simulink model "SUB_IoControl"  (R2018b)
settings: Solver=VariableStepDiscrete  StartTime=0.0  StopTime=10  RelTol=1e-3
PreLoadFcn:
  | if(exist('MBDS_ModelCallback', 'file'))
  |    MBDS_ModelCallback('PreLoad');
  | end
PostLoadFcn:
  | if(exist('MBDS_ModelCallback', 'file'))
  |    MBDS_ModelCallback('PostLoad');
  | end
InitFcn:
  | if(exist('MBDS_ModelCallback', 'file'))
  |    MBDS_ModelCallback('Init');
  | end
StartFcn:
  | if(exist('MBDS_ModelCallback', 'file'))
  |    MBDS_ModelCallback('Start');
  | end
StopFcn:
  | if(exist('MBDS_ModelCallback', 'file'))
  |    MBDS_ModelCallback('Stop');
  | end
undefined symbols (not defined in the file): sigbuilder_block
libraries: KIBES_Signal x742, MBDS_Modules x38, simulink x1
(part 2 of 8)

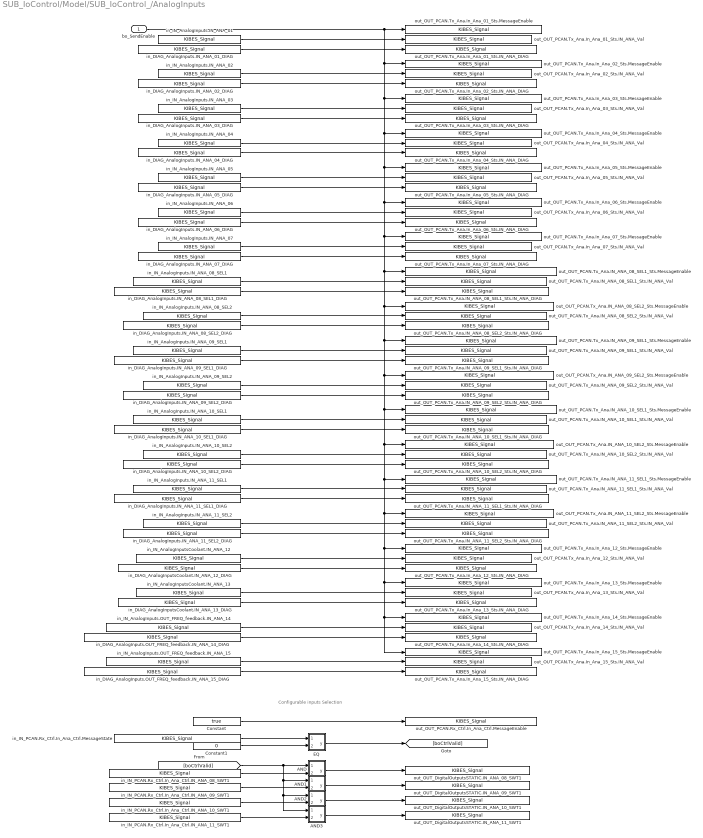
== system SUB_IoControl/Model/SUB_IoControl_/AnalogInputs ==
  note: Configurable inputs Selection
  bo_SendEnable : Inport
  AND : Subsystem  InitFcn=|  mask(AND){MBDS_LibraryBlock=on, BitwiseMode=off, Inputs=2, UseBitMask=off, BitMask='A7', OutDataTypeStr=Inherit: Inherit via back propagation, MBDS_BlockVersion=08.20.02}
      | if(exist('MBDS_BlockCallback', 'file'))
      |    MBDS_BlockCallback('Update', gcb);
      | end
      mask prompts: MBDS_LibraryBlock "MBDS library block"; BitwiseMode "Use 'bitwise' mode"; Inputs "Number of input ports:"; UseBitMask "Use bit mask"; BitMask "Bit mask:"; OutDataTypeStr "Output data type:"; MBDS_BlockVersion "Version:"
      mask help: Logical or bitwise AND operator. For multiple inputs, operators are applied across the inputs. For a single input, operators are applied across the input vector. In bitwise mode a bit mask can be applied onto single input signals.
      mask init: same as SUB_IoControl/Outputs/AnalyseOutputs/And
      mask Help: eval(['open([workdir(''library_dir:''),''\Blockset\help\'',get_param(gcb,''MaskType''),''.html''])'])
      mask Callback BitwiseMode:
      | if(exist('MBDS_BlockCallback', 'file'))
      |    MBDS_BlockCallback('BitwiseMode', gcb);
      | end
      mask Callback Inputs:
      | if(exist('MBDS_BlockCallback', 'file'))
      |    MBDS_BlockCallback('Inputs', gcb);
      | end
      mask Callback UseBitMask:
      | if(exist('MBDS_BlockCallback', 'file'))
      |    MBDS_BlockCallback('UseBitMask', gcb);
      | end
      mask Callback BitMask:
      | if(exist('MBDS_BlockCallback', 'file'))
      |    MBDS_BlockCallback('BitMask', gcb);
      | end
      mask TypeOptions OutDataTypeStr: Inherit: Inherit via back propagation | int8 | uint8 | int16 | uint16 | int32 | uint32 | boolean
      mask Callback OutDataTypeStr:
      | % Adopt Value
      | if(exist('MBDS_BlockCallback', 'file'))
      |    MBDS_BlockCallback('OutDataTypeStr', gcb);
      | end
      mask DialogControl ParameterTabVar0 Prompt: Main
      mask DialogControl ParameterTabVar01 Prompt: Signal Attributes
      mask DialogControl ParameterTabVar012 Prompt: Version
      mask Display:
      | % Show icon or block text
      | if(UseBitMask)
      |    if(isnumeric(BitMask))
      |       BitMaskString = ['0x',dec2hex(floor(BitMask))];
      |    elseif(ischar(BitMask))
      |       BitMaskString = ['0x',upper(BitMask)];
      |    else
      |       BitMaskString = '???';
      |    end
      |    disp(sprintf(['AND\n', BitMaskString]))
      | else
      |    disp('AND')
      | end
  AND1 : Subsystem  InitFcn=|  mask(AND){MBDS_LibraryBlock=on, BitwiseMode=off, Inputs=2, UseBitMask=off, BitMask='A7', OutDataTypeStr=Inherit: Inherit via back propagation, MBDS_BlockVersion=08.20.02}
      | if(exist('MBDS_BlockCallback', 'file'))
      |    MBDS_BlockCallback('Update', gcb);
      | end
      mask prompts: MBDS_LibraryBlock "MBDS library block"; BitwiseMode "Use 'bitwise' mode"; Inputs "Number of input ports:"; UseBitMask "Use bit mask"; BitMask "Bit mask:"; OutDataTypeStr "Output data type:"; MBDS_BlockVersion "Version:"
      mask help: Logical or bitwise AND operator. For multiple inputs, operators are applied across the inputs. For a single input, operators are applied across the input vector. In bitwise mode a bit mask can be applied onto single input signals.
      mask init: same as SUB_IoControl/Outputs/AnalyseOutputs/And
      mask Help: eval(['open([workdir(''library_dir:''),''\Blockset\help\'',get_param(gcb,''MaskType''),''.html''])'])
      mask Callback BitwiseMode:
      | if(exist('MBDS_BlockCallback', 'file'))
      |    MBDS_BlockCallback('BitwiseMode', gcb);
      | end
      mask Callback Inputs:
      | if(exist('MBDS_BlockCallback', 'file'))
      |    MBDS_BlockCallback('Inputs', gcb);
      | end
      mask Callback UseBitMask:
      | if(exist('MBDS_BlockCallback', 'file'))
      |    MBDS_BlockCallback('UseBitMask', gcb);
      | end
      mask Callback BitMask:
      | if(exist('MBDS_BlockCallback', 'file'))
      |    MBDS_BlockCallback('BitMask', gcb);
      | end
      mask TypeOptions OutDataTypeStr: Inherit: Inherit via back propagation | int8 | uint8 | int16 | uint16 | int32 | uint32 | boolean
      mask Callback OutDataTypeStr:
      | % Adopt Value
      | if(exist('MBDS_BlockCallback', 'file'))
      |    MBDS_BlockCallback('OutDataTypeStr', gcb);
      | end
      mask DialogControl ParameterTabVar0 Prompt: Main
      mask DialogControl ParameterTabVar01 Prompt: Signal Attributes
      mask DialogControl ParameterTabVar012 Prompt: Version
      mask Display:
      | % Show icon or block text
      | if(UseBitMask)
      |    if(isnumeric(BitMask))
      |       BitMaskString = ['0x',dec2hex(floor(BitMask))];
      |    elseif(ischar(BitMask))
      |       BitMaskString = ['0x',upper(BitMask)];
      |    else
      |       BitMaskString = '???';
      |    end
      |    disp(sprintf(['AND\n', BitMaskString]))
      | else
      |    disp('AND')
      | end
  AND2 : Subsystem  InitFcn=|  mask(AND){MBDS_LibraryBlock=on, BitwiseMode=off, Inputs=2, UseBitMask=off, BitMask='A7', OutDataTypeStr=Inherit: Inherit via back propagation, MBDS_BlockVersion=08.20.02}
      | if(exist('MBDS_BlockCallback', 'file'))
      |    MBDS_BlockCallback('Update', gcb);
      | end
      mask prompts: MBDS_LibraryBlock "MBDS library block"; BitwiseMode "Use 'bitwise' mode"; Inputs "Number of input ports:"; UseBitMask "Use bit mask"; BitMask "Bit mask:"; OutDataTypeStr "Output data type:"; MBDS_BlockVersion "Version:"
      mask help: Logical or bitwise AND operator. For multiple inputs, operators are applied across the inputs. For a single input, operators are applied across the input vector. In bitwise mode a bit mask can be applied onto single input signals.
      mask init: same as SUB_IoControl/Outputs/AnalyseOutputs/And
      mask Help: eval(['open([workdir(''library_dir:''),''\Blockset\help\'',get_param(gcb,''MaskType''),''.html''])'])
      mask Callback BitwiseMode:
      | if(exist('MBDS_BlockCallback', 'file'))
      |    MBDS_BlockCallback('BitwiseMode', gcb);
      | end
      mask Callback Inputs:
      | if(exist('MBDS_BlockCallback', 'file'))
      |    MBDS_BlockCallback('Inputs', gcb);
      | end
      mask Callback UseBitMask:
      | if(exist('MBDS_BlockCallback', 'file'))
      |    MBDS_BlockCallback('UseBitMask', gcb);
      | end
      mask Callback BitMask:
      | if(exist('MBDS_BlockCallback', 'file'))
      |    MBDS_BlockCallback('BitMask', gcb);
      | end
      mask TypeOptions OutDataTypeStr: Inherit: Inherit via back propagation | int8 | uint8 | int16 | uint16 | int32 | uint32 | boolean
      mask Callback OutDataTypeStr:
      | % Adopt Value
      | if(exist('MBDS_BlockCallback', 'file'))
      |    MBDS_BlockCallback('OutDataTypeStr', gcb);
      | end
      mask DialogControl ParameterTabVar0 Prompt: Main
      mask DialogControl ParameterTabVar01 Prompt: Signal Attributes
      mask DialogControl ParameterTabVar012 Prompt: Version
      mask Display:
      | % Show icon or block text
      | if(UseBitMask)
      |    if(isnumeric(BitMask))
      |       BitMaskString = ['0x',dec2hex(floor(BitMask))];
      |    elseif(ischar(BitMask))
      |       BitMaskString = ['0x',upper(BitMask)];
      |    else
      |       BitMaskString = '???';
      |    end
      |    disp(sprintf(['AND\n', BitMaskString]))
      | else
      |    disp('AND')
      | end
  AND3 : Subsystem  InitFcn=|  mask(AND){MBDS_LibraryBlock=on, BitwiseMode=off, Inputs=2, UseBitMask=off, BitMask='A7', OutDataTypeStr=Inherit: Inherit via back propagation, MBDS_BlockVersion=08.20.02}
      | if(exist('MBDS_BlockCallback', 'file'))
      |    MBDS_BlockCallback('Update', gcb);
      | end
      mask prompts: MBDS_LibraryBlock "MBDS library block"; BitwiseMode "Use 'bitwise' mode"; Inputs "Number of input ports:"; UseBitMask "Use bit mask"; BitMask "Bit mask:"; OutDataTypeStr "Output data type:"; MBDS_BlockVersion "Version:"
      mask help: Logical or bitwise AND operator. For multiple inputs, operators are applied across the inputs. For a single input, operators are applied across the input vector. In bitwise mode a bit mask can be applied onto single input signals.
      mask init: same as SUB_IoControl/Outputs/AnalyseOutputs/And
      mask Help: eval(['open([workdir(''library_dir:''),''\Blockset\help\'',get_param(gcb,''MaskType''),''.html''])'])
      mask Callback BitwiseMode:
      | if(exist('MBDS_BlockCallback', 'file'))
      |    MBDS_BlockCallback('BitwiseMode', gcb);
      | end
      mask Callback Inputs:
      | if(exist('MBDS_BlockCallback', 'file'))
      |    MBDS_BlockCallback('Inputs', gcb);
      | end
      mask Callback UseBitMask:
      | if(exist('MBDS_BlockCallback', 'file'))
      |    MBDS_BlockCallback('UseBitMask', gcb);
      | end
      mask Callback BitMask:
      | if(exist('MBDS_BlockCallback', 'file'))
      |    MBDS_BlockCallback('BitMask', gcb);
      | end
      mask TypeOptions OutDataTypeStr: Inherit: Inherit via back propagation | int8 | uint8 | int16 | uint16 | int32 | uint32 | boolean
      mask Callback OutDataTypeStr:
      | % Adopt Value
      | if(exist('MBDS_BlockCallback', 'file'))
      |    MBDS_BlockCallback('OutDataTypeStr', gcb);
      | end
      mask DialogControl ParameterTabVar0 Prompt: Main
      mask DialogControl ParameterTabVar01 Prompt: Signal Attributes
      mask DialogControl ParameterTabVar012 Prompt: Version
      mask Display:
      | % Show icon or block text
      | if(UseBitMask)
      |    if(isnumeric(BitMask))
      |       BitMaskString = ['0x',dec2hex(floor(BitMask))];
      |    elseif(ischar(BitMask))
      |       BitMaskString = ['0x',upper(BitMask)];
      |    else
      |       BitMaskString = '???';
      |    end
      |    disp(sprintf(['AND\n', BitMaskString]))
      | else
      |    disp('AND')
      | end
  Constant : Constant  InitFcn=|  Value=true  OutDataTypeStr=boolean
      | if(exist('MBDS_BlockCallback', 'file'))
      |    MBDS_BlockCallback('Update', gcb);  
      | end
  Constant1 : Constant  InitFcn=|  Value=0  OutDataTypeStr=uint16
      | if(exist('MBDS_BlockCallback', 'file'))
      |    MBDS_BlockCallback('Update', gcb);  
      | end
  EQ : Subsystem  InitFcn=|  mask(EQ){MBDS_LibraryBlock=on, InputSameDT=on, MBDS_BlockVersion=08.20.02}
      | if(exist('MBDS_BlockCallback', 'file'))
      |    MBDS_BlockCallback('Update', gcb);
      | end
      mask prompts: MBDS_LibraryBlock "MBDS library block"; InputSameDT "Require all inputs to have the same data type"; MBDS_BlockVersion "Block version:"
      mask help: The block compares if both input signals are equal.
      mask init: same as SUB_IoControl/Outputs/AnalyseOutputs/And
      mask Help: eval(['open([workdir(''library_dir:''),''\Blockset\help\'',get_param(gcb,''MaskType''),''.html''])'])
      mask Callback InputSameDT:
      | % Adopt value
      | if(exist('MBDS_BlockCallback', 'file'))
      |    MBDS_BlockCallback('InputSameDT', gcb);
      | end
      mask DialogControl ParameterTabVar0 Prompt: Signal Attributes
      mask DialogControl ParameterTabVar01 Prompt: Version
      mask Display:
      | % Show icon or block text
      | if(exist('MBDS_BlockCallback', 'file'))
      |    image(imread('EQ.tif','tif'),[0.35,0.35,0.355,0.25])
      |    disp('')
      | else
      |    disp(sprintf('=='));
      | end
  in_DIAG_AnalogInputs.IN_ANA_01_DIAG : KIBES_Signal/KIBES_Signal  MBDS_LibraryBlock=on  DatabaseKey=635  SignalName=DIAG_AnalogInputs.IN_ANA_01_DIAG  SymbolName=DIAG_AnalogInputs_IN_ANA_01_DIAG_000635  DataType=uint16  Init=1  Slope=1  Bias=0  DataSize=1  fpDataType=uint16  BlockIOType=Inport  DeviceType=0
  in_DIAG_AnalogInputs.IN_ANA_02_DIAG : KIBES_Signal/KIBES_Signal  MBDS_LibraryBlock=on  DatabaseKey=626  SignalName=DIAG_AnalogInputs.IN_ANA_02_DIAG  SymbolName=DIAG_AnalogInputs_IN_ANA_02_DIAG_000626  DataType=uint16  Init=1  Slope=1  Bias=0  DataSize=1  fpDataType=uint16  BlockIOType=Inport  DeviceType=0
  in_DIAG_AnalogInputs.IN_ANA_03_DIAG : KIBES_Signal/KIBES_Signal  MBDS_LibraryBlock=on  DatabaseKey=628  SignalName=DIAG_AnalogInputs.IN_ANA_03_DIAG  SymbolName=DIAG_AnalogInputs_IN_ANA_03_DIAG_000628  DataType=uint16  Init=1  Slope=1  Bias=0  DataSize=1  fpDataType=uint16  BlockIOType=Inport  DeviceType=0
  in_DIAG_AnalogInputs.IN_ANA_04_DIAG : KIBES_Signal/KIBES_Signal  MBDS_LibraryBlock=on  DatabaseKey=630  SignalName=DIAG_AnalogInputs.IN_ANA_04_DIAG  SymbolName=DIAG_AnalogInputs_IN_ANA_04_DIAG_000630  DataType=uint16  Init=1  Slope=1  Bias=0  DataSize=1  fpDataType=uint16  BlockIOType=Inport  DeviceType=0
  in_DIAG_AnalogInputs.IN_ANA_05_DIAG : KIBES_Signal/KIBES_Signal  MBDS_LibraryBlock=on  DatabaseKey=632  SignalName=DIAG_AnalogInputs.IN_ANA_05_DIAG  SymbolName=DIAG_AnalogInputs_IN_ANA_05_DIAG_000632  DataType=uint16  Init=1  Slope=1  Bias=0  DataSize=1  fpDataType=uint16  BlockIOType=Inport  DeviceType=0
  in_DIAG_AnalogInputs.IN_ANA_06_DIAG : KIBES_Signal/KIBES_Signal  MBDS_LibraryBlock=on  DatabaseKey=636  SignalName=DIAG_AnalogInputs.IN_ANA_06_DIAG  SymbolName=DIAG_AnalogInputs_IN_ANA_06_DIAG_000636  DataType=uint16  Init=1  Slope=1  Bias=0  DataSize=1  fpDataType=uint16  BlockIOType=Inport  DeviceType=0
  in_DIAG_AnalogInputs.IN_ANA_07_DIAG : KIBES_Signal/KIBES_Signal  MBDS_LibraryBlock=on  DatabaseKey=638  SignalName=DIAG_AnalogInputs.IN_ANA_07_DIAG  SymbolName=DIAG_AnalogInputs_IN_ANA_07_DIAG_000638  DataType=uint16  Init=1  Slope=1  Bias=0  DataSize=1  fpDataType=uint16  BlockIOType=Inport  DeviceType=0
  in_DIAG_AnalogInputs.IN_ANA_08_SEL1_DIAG : KIBES_Signal/KIBES_Signal  MBDS_LibraryBlock=on  DatabaseKey=640  SignalName=DIAG_AnalogInputs.IN_ANA_08_SEL1_DIAG  SymbolName=DIAG_AnalogInputs_IN_ANA_08_SEL1_DIAG_000640  DataType=uint16  Init=1  Slope=1  Bias=0  DataSize=1  fpDataType=uint16  BlockIOType=Inport  DeviceType=0
  in_DIAG_AnalogInputs.IN_ANA_08_SEL2_DIAG : KIBES_Signal/KIBES_Signal  MBDS_LibraryBlock=on  DatabaseKey=2275  SignalName=DIAG_AnalogInputs.IN_ANA_08_SEL2_DIAG  SymbolName=DIAG_AnalogInputs_IN_ANA_08_SEL2_DIAG_002275  DataType=uint16  Init=1  Slope=1  Bias=0  DataSize=1  fpDataType=uint16  BlockIOType=Inport  DeviceType=0
  in_DIAG_AnalogInputs.IN_ANA_09_SEL1_DIAG : KIBES_Signal/KIBES_Signal  MBDS_LibraryBlock=on  DatabaseKey=642  SignalName=DIAG_AnalogInputs.IN_ANA_09_SEL1_DIAG  SymbolName=DIAG_AnalogInputs_IN_ANA_09_SEL1_DIAG_000642  DataType=uint16  Init=1  Slope=1  Bias=0  DataSize=1  fpDataType=uint16  BlockIOType=Inport  DeviceType=0
  in_DIAG_AnalogInputs.IN_ANA_09_SEL2_DIAG : KIBES_Signal/KIBES_Signal  MBDS_LibraryBlock=on  DatabaseKey=2277  SignalName=DIAG_AnalogInputs.IN_ANA_09_SEL2_DIAG  SymbolName=DIAG_AnalogInputs_IN_ANA_09_SEL2_DIAG_002277  DataType=uint16  Init=1  Slope=1  Bias=0  DataSize=1  fpDataType=uint16  BlockIOType=Inport  DeviceType=0
  in_DIAG_AnalogInputs.IN_ANA_10_SEL1_DIAG : KIBES_Signal/KIBES_Signal  MBDS_LibraryBlock=on  DatabaseKey=644  SignalName=DIAG_AnalogInputs.IN_ANA_10_SEL1_DIAG  SymbolName=DIAG_AnalogInputs_IN_ANA_10_SEL1_DIAG_000644  DataType=uint16  Init=1  Slope=1  Bias=0  DataSize=1  fpDataType=uint16  BlockIOType=Inport  DeviceType=0
  in_DIAG_AnalogInputs.IN_ANA_10_SEL2_DIAG : KIBES_Signal/KIBES_Signal  MBDS_LibraryBlock=on  DatabaseKey=2279  SignalName=DIAG_AnalogInputs.IN_ANA_10_SEL2_DIAG  SymbolName=DIAG_AnalogInputs_IN_ANA_10_SEL2_DIAG_002279  DataType=uint16  Init=1  Slope=1  Bias=0  DataSize=1  fpDataType=uint16  BlockIOType=Inport  DeviceType=0
  in_DIAG_AnalogInputs.IN_ANA_11_SEL1_DIAG : KIBES_Signal/KIBES_Signal  MBDS_LibraryBlock=on  DatabaseKey=646  SignalName=DIAG_AnalogInputs.IN_ANA_11_SEL1_DIAG  SymbolName=DIAG_AnalogInputs_IN_ANA_11_SEL1_DIAG_000646  DataType=uint16  Init=1  Slope=1  Bias=0  DataSize=1  fpDataType=uint16  BlockIOType=Inport  DeviceType=0
  in_DIAG_AnalogInputs.IN_ANA_11_SEL2_DIAG : KIBES_Signal/KIBES_Signal  MBDS_LibraryBlock=on  DatabaseKey=2281  SignalName=DIAG_AnalogInputs.IN_ANA_11_SEL2_DIAG  SymbolName=DIAG_AnalogInputs_IN_ANA_11_SEL2_DIAG_002281  DataType=uint16  Init=1  Slope=1  Bias=0  DataSize=1  fpDataType=uint16  BlockIOType=Inport  DeviceType=0
  in_DIAG_AnalogInputs.OUT_FREQ_feedback.IN_ANA_14_DIAG : KIBES_Signal/KIBES_Signal  MBDS_LibraryBlock=on  DatabaseKey=697  SignalName=DIAG_AnalogInputs.OUT_FREQ_feedback.IN_ANA_14_DIAG  SymbolName=DIAG_AnalogInputs_OUT_FREQ_feedback_IN_ANA_14_DIAG_000697  DataType=uint16  Init=1  Slope=1  Bias=0  DataSize=1  fpDataType=uint16  BlockIOType=Inport  DeviceType=0
  in_DIAG_AnalogInputs.OUT_FREQ_feedback.IN_ANA_15_DIAG : KIBES_Signal/KIBES_Signal  MBDS_LibraryBlock=on  DatabaseKey=699  SignalName=DIAG_AnalogInputs.OUT_FREQ_feedback.IN_ANA_15_DIAG  SymbolName=DIAG_AnalogInputs_OUT_FREQ_feedback_IN_ANA_15_DIAG_000699  DataType=uint16  Init=1  Slope=1  Bias=0  DataSize=1  fpDataType=uint16  BlockIOType=Inport  DeviceType=0
  in_DIAG_AnalogInputsCoolant.IN_ANA_12_DIAG : KIBES_Signal/KIBES_Signal  MBDS_LibraryBlock=on  DatabaseKey=693  SignalName=DIAG_AnalogInputsCoolant.IN_ANA_12_DIAG  SymbolName=DIAG_AnalogInputsCoolant_IN_ANA_12_DIAG_000693  DataType=uint16  Init=1  Slope=1  Bias=0  DataSize=1  fpDataType=uint16  BlockIOType=Inport  DeviceType=0
  in_DIAG_AnalogInputsCoolant.IN_ANA_13_DIAG : KIBES_Signal/KIBES_Signal  MBDS_LibraryBlock=on  DatabaseKey=695  SignalName=DIAG_AnalogInputsCoolant.IN_ANA_13_DIAG  SymbolName=DIAG_AnalogInputsCoolant_IN_ANA_13_DIAG_000695  DataType=uint16  Init=1  Slope=1  Bias=0  DataSize=1  fpDataType=uint16  BlockIOType=Inport  DeviceType=0
  in_IN_AnalogInputs.IN_ANA_01 : KIBES_Signal/KIBES_Signal  MBDS_LibraryBlock=on  DatabaseKey=634  SignalName=IN_AnalogInputs.IN_ANA_01  SymbolName=IN_AnalogInputs_IN_ANA_01_000634  DataType=uint32  Init=0  Slope=1  Bias=0  DataSize=1  fpDataType=uint32  BlockIOType=Inport  DeviceType=0
  in_IN_AnalogInputs.IN_ANA_02 : KIBES_Signal/KIBES_Signal  MBDS_LibraryBlock=on  DatabaseKey=625  SignalName=IN_AnalogInputs.IN_ANA_02  SymbolName=IN_AnalogInputs_IN_ANA_02_000625  DataType=uint32  Init=0  Slope=1  Bias=0  DataSize=1  fpDataType=uint32  BlockIOType=Inport  DeviceType=0
  in_IN_AnalogInputs.IN_ANA_03 : KIBES_Signal/KIBES_Signal  MBDS_LibraryBlock=on  DatabaseKey=627  SignalName=IN_AnalogInputs.IN_ANA_03  SymbolName=IN_AnalogInputs_IN_ANA_03_000627  DataType=uint32  Init=0  Slope=1  Bias=0  DataSize=1  fpDataType=uint32  BlockIOType=Inport  DeviceType=0
  in_IN_AnalogInputs.IN_ANA_04 : KIBES_Signal/KIBES_Signal  MBDS_LibraryBlock=on  DatabaseKey=629  SignalName=IN_AnalogInputs.IN_ANA_04  SymbolName=IN_AnalogInputs_IN_ANA_04_000629  DataType=uint32  Init=0  Slope=1  Bias=0  DataSize=1  fpDataType=uint32  BlockIOType=Inport  DeviceType=0
  in_IN_AnalogInputs.IN_ANA_05 : KIBES_Signal/KIBES_Signal  MBDS_LibraryBlock=on  DatabaseKey=631  SignalName=IN_AnalogInputs.IN_ANA_05  SymbolName=IN_AnalogInputs_IN_ANA_05_000631  DataType=uint32  Init=0  Slope=1  Bias=0  DataSize=1  fpDataType=uint32  BlockIOType=Inport  DeviceType=0
  in_IN_AnalogInputs.IN_ANA_06 : KIBES_Signal/KIBES_Signal  MBDS_LibraryBlock=on  DatabaseKey=633  SignalName=IN_AnalogInputs.IN_ANA_06  SymbolName=IN_AnalogInputs_IN_ANA_06_000633  DataType=uint32  Init=0  Slope=1  Bias=0  DataSize=1  fpDataType=uint32  BlockIOType=Inport  DeviceType=0
  in_IN_AnalogInputs.IN_ANA_07 : KIBES_Signal/KIBES_Signal  MBDS_LibraryBlock=on  DatabaseKey=637  SignalName=IN_AnalogInputs.IN_ANA_07  SymbolName=IN_AnalogInputs_IN_ANA_07_000637  DataType=uint32  Init=0  Slope=1  Bias=0  DataSize=1  fpDataType=uint32  BlockIOType=Inport  DeviceType=0
  in_IN_AnalogInputs.IN_ANA_08_SEL1 : KIBES_Signal/KIBES_Signal  MBDS_LibraryBlock=on  DatabaseKey=639  SignalName=IN_AnalogInputs.IN_ANA_08_SEL1  SymbolName=IN_AnalogInputs_IN_ANA_08_SEL1_000639  DataType=uint32  Init=0  Slope=1  Bias=0  DataSize=1  fpDataType=uint32  BlockIOType=Inport  DeviceType=0
  in_IN_AnalogInputs.IN_ANA_08_SEL2 : KIBES_Signal/KIBES_Signal  MBDS_LibraryBlock=on  DatabaseKey=2274  SignalName=IN_AnalogInputs.IN_ANA_08_SEL2  SymbolName=IN_AnalogInputs_IN_ANA_08_SEL2_002274  DataType=uint32  Init=0  Slope=1  Bias=0  DataSize=1  fpDataType=uint32  BlockIOType=Inport  DeviceType=0
  in_IN_AnalogInputs.IN_ANA_09_SEL1 : KIBES_Signal/KIBES_Signal  MBDS_LibraryBlock=on  DatabaseKey=641  SignalName=IN_AnalogInputs.IN_ANA_09_SEL1  SymbolName=IN_AnalogInputs_IN_ANA_09_SEL1_000641  DataType=uint32  Init=0  Slope=1  Bias=0  DataSize=1  fpDataType=uint32  BlockIOType=Inport  DeviceType=0
  in_IN_AnalogInputs.IN_ANA_09_SEL2 : KIBES_Signal/KIBES_Signal  MBDS_LibraryBlock=on  DatabaseKey=2276  SignalName=IN_AnalogInputs.IN_ANA_09_SEL2  SymbolName=IN_AnalogInputs_IN_ANA_09_SEL2_002276  DataType=uint32  Init=0  Slope=1  Bias=0  DataSize=1  fpDataType=uint32  BlockIOType=Inport  DeviceType=0
  in_IN_AnalogInputs.IN_ANA_10_SEL1 : KIBES_Signal/KIBES_Signal  MBDS_LibraryBlock=on  DatabaseKey=643  SignalName=IN_AnalogInputs.IN_ANA_10_SEL1  SymbolName=IN_AnalogInputs_IN_ANA_10_SEL1_000643  DataType=uint32  Init=0  Slope=1  Bias=0  DataSize=1  fpDataType=uint32  BlockIOType=Inport  DeviceType=0
  in_IN_AnalogInputs.IN_ANA_10_SEL2 : KIBES_Signal/KIBES_Signal  MBDS_LibraryBlock=on  DatabaseKey=2278  SignalName=IN_AnalogInputs.IN_ANA_10_SEL2  SymbolName=IN_AnalogInputs_IN_ANA_10_SEL2_002278  DataType=uint32  Init=0  Slope=1  Bias=0  DataSize=1  fpDataType=uint32  BlockIOType=Inport  DeviceType=0
  in_IN_AnalogInputs.IN_ANA_11_SEL1 : KIBES_Signal/KIBES_Signal  MBDS_LibraryBlock=on  DatabaseKey=645  SignalName=IN_AnalogInputs.IN_ANA_11_SEL1  SymbolName=IN_AnalogInputs_IN_ANA_11_SEL1_000645  DataType=uint32  Init=0  Slope=1  Bias=0  DataSize=1  fpDataType=uint32  BlockIOType=Inport  DeviceType=0
  in_IN_AnalogInputs.IN_ANA_11_SEL2 : KIBES_Signal/KIBES_Signal  MBDS_LibraryBlock=on  DatabaseKey=2280  SignalName=IN_AnalogInputs.IN_ANA_11_SEL2  SymbolName=IN_AnalogInputs_IN_ANA_11_SEL2_002280  DataType=uint32  Init=0  Slope=1  Bias=0  DataSize=1  fpDataType=uint32  BlockIOType=Inport  DeviceType=0
  in_IN_AnalogInputs.OUT_FREQ_feedback.IN_ANA_14 : KIBES_Signal/KIBES_Signal  MBDS_LibraryBlock=on  DatabaseKey=696  SignalName=IN_AnalogInputs.OUT_FREQ_feedback.IN_ANA_14  SymbolName=IN_AnalogInputs_OUT_FREQ_feedback_IN_ANA_14_000696  DataType=uint32  Init=0  Slope=1  Bias=0  DataSize=1  fpDataType=uint32  BlockIOType=Inport  DeviceType=0
  in_IN_AnalogInputs.OUT_FREQ_feedback.IN_ANA_15 : KIBES_Signal/KIBES_Signal  MBDS_LibraryBlock=on  DatabaseKey=698  SignalName=IN_AnalogInputs.OUT_FREQ_feedback.IN_ANA_15  SymbolName=IN_AnalogInputs_OUT_FREQ_feedback_IN_ANA_15_000698  DataType=uint32  Init=0  Slope=1  Bias=0  DataSize=1  fpDataType=uint32  BlockIOType=Inport  DeviceType=0
  in_IN_AnalogInputsCoolant.IN_ANA_12 : KIBES_Signal/KIBES_Signal  MBDS_LibraryBlock=on  DatabaseKey=692  SignalName=IN_AnalogInputsCoolant.IN_ANA_12  SymbolName=IN_AnalogInputsCoolant_IN_ANA_12_000692  DataType=uint32  Init=0  Slope=1  Bias=0  DataSize=1  fpDataType=uint32  BlockIOType=Inport  DeviceType=0
  in_IN_AnalogInputsCoolant.IN_ANA_13 : KIBES_Signal/KIBES_Signal  MBDS_LibraryBlock=on  DatabaseKey=694  SignalName=IN_AnalogInputsCoolant.IN_ANA_13  SymbolName=IN_AnalogInputsCoolant_IN_ANA_13_000694  DataType=uint32  Init=0  Slope=1  Bias=0  DataSize=1  fpDataType=uint32  BlockIOType=Inport  DeviceType=0
  in_IN_PCAN.Rx_Ctrl.In_Ana_Ctrl.IN_ANA_08_SWT1 : KIBES_Signal/KIBES_Signal  MBDS_LibraryBlock=on  DatabaseKey=2163  SignalName=IN_PCAN.Rx_Ctrl.In_Ana_Ctrl.IN_ANA_08_SWT1  SymbolName=IN_PCAN_Rx_Ctrl_In_Ana_Ctrl_IN_ANA_08_SWT1_002163  DataType=boolean  Init=0  Slope=1  Bias=0  DataSize=1  fpDataType=boolean  BlockIOType=Inport  DeviceType=0
  in_IN_PCAN.Rx_Ctrl.In_Ana_Ctrl.IN_ANA_09_SWT1 : KIBES_Signal/KIBES_Signal  MBDS_LibraryBlock=on  DatabaseKey=2164  SignalName=IN_PCAN.Rx_Ctrl.In_Ana_Ctrl.IN_ANA_09_SWT1  SymbolName=IN_PCAN_Rx_Ctrl_In_Ana_Ctrl_IN_ANA_09_SWT1_002164  DataType=boolean  Init=0  Slope=1  Bias=0  DataSize=1  fpDataType=boolean  BlockIOType=Inport  DeviceType=0
  in_IN_PCAN.Rx_Ctrl.In_Ana_Ctrl.IN_ANA_10_SWT1 : KIBES_Signal/KIBES_Signal  MBDS_LibraryBlock=on  DatabaseKey=2165  SignalName=IN_PCAN.Rx_Ctrl.In_Ana_Ctrl.IN_ANA_10_SWT1  SymbolName=IN_PCAN_Rx_Ctrl_In_Ana_Ctrl_IN_ANA_10_SWT1_002165  DataType=boolean  Init=0  Slope=1  Bias=0  DataSize=1  fpDataType=boolean  BlockIOType=Inport  DeviceType=0
  in_IN_PCAN.Rx_Ctrl.In_Ana_Ctrl.IN_ANA_11_SWT1 : KIBES_Signal/KIBES_Signal  MBDS_LibraryBlock=on  DatabaseKey=2166  SignalName=IN_PCAN.Rx_Ctrl.In_Ana_Ctrl.IN_ANA_11_SWT1  SymbolName=IN_PCAN_Rx_Ctrl_In_Ana_Ctrl_IN_ANA_11_SWT1_002166  DataType=boolean  Init=0  Slope=1  Bias=0  DataSize=1  fpDataType=boolean  BlockIOType=Inport  DeviceType=0
  in_IN_PCAN.Rx_Ctrl.In_Ana_Ctrl.MessageState : KIBES_Signal/KIBES_Signal  MBDS_LibraryBlock=on  DatabaseKey=2168  SignalName=IN_PCAN.Rx_Ctrl.In_Ana_Ctrl.MessageState  SymbolName=IN_PCAN_Rx_Ctrl_In_Ana_Ctrl_MessageState_002168  DataType=uint16  Init=0  Slope=1  Bias=0  DataSize=1  fpDataType=uint16  BlockIOType=Inport  DeviceType=0
  out_OUT_DigitalOutputsSTATIC.IN_ANA_08_SWT1 : KIBES_Signal/KIBES_Signal  MBDS_LibraryBlock=on  DatabaseKey=2285  SignalName=OUT_DigitalOutputsSTATIC.IN_ANA_08_SWT1  SymbolName=OUT_DigitalOutputsSTATIC_IN_ANA_08_SWT1_002285  DataType=boolean  Init=0  Slope=1  Bias=0  DataSize=1  fpDataType=boolean  BlockIOType=Outport  DeviceType=0
  out_OUT_DigitalOutputsSTATIC.IN_ANA_09_SWT1 : KIBES_Signal/KIBES_Signal  MBDS_LibraryBlock=on  DatabaseKey=2286  SignalName=OUT_DigitalOutputsSTATIC.IN_ANA_09_SWT1  SymbolName=OUT_DigitalOutputsSTATIC_IN_ANA_09_SWT1_002286  DataType=boolean  Init=0  Slope=1  Bias=0  DataSize=1  fpDataType=boolean  BlockIOType=Outport  DeviceType=0
  out_OUT_DigitalOutputsSTATIC.IN_ANA_10_SWT1 : KIBES_Signal/KIBES_Signal  MBDS_LibraryBlock=on  DatabaseKey=2287  SignalName=OUT_DigitalOutputsSTATIC.IN_ANA_10_SWT1  SymbolName=OUT_DigitalOutputsSTATIC_IN_ANA_10_SWT1_002287  DataType=boolean  Init=0  Slope=1  Bias=0  DataSize=1  fpDataType=boolean  BlockIOType=Outport  DeviceType=0
  out_OUT_DigitalOutputsSTATIC.IN_ANA_11_SWT1 : KIBES_Signal/KIBES_Signal  MBDS_LibraryBlock=on  DatabaseKey=2288  SignalName=OUT_DigitalOutputsSTATIC.IN_ANA_11_SWT1  SymbolName=OUT_DigitalOutputsSTATIC_IN_ANA_11_SWT1_002288  DataType=boolean  Init=0  Slope=1  Bias=0  DataSize=1  fpDataType=boolean  BlockIOType=Outport  DeviceType=0
  out_OUT_PCAN.Rx_Ctrl.In_Ana_Ctrl.MessageEnable : KIBES_Signal/KIBES_Signal  MBDS_LibraryBlock=on  DatabaseKey=2167  SignalName=OUT_PCAN.Rx_Ctrl.In_Ana_Ctrl.MessageEnable  SymbolName=OUT_PCAN_Rx_Ctrl_In_Ana_Ctrl_MessageEnable_002167  DataType=boolean  Init=0  Slope=1  Bias=0  DataSize=1  fpDataType=boolean  BlockIOType=Outport  DeviceType=0
  out_OUT_PCAN.Tx_Ana.IN_ANA_08_SEL1_Sts.IN_ANA_DIAG : KIBES_Signal/KIBES_Signal  MBDS_LibraryBlock=on  DatabaseKey=2139  SignalName=OUT_PCAN.Tx_Ana.IN_ANA_08_SEL1_Sts.IN_ANA_DIAG  SymbolName=OUT_PCAN_Tx_Ana_IN_ANA_08_SEL1_Sts_IN_ANA_DIAG_002139  DataType=uint16  Init=0  Slope=1  Bias=0  DataSize=1  fpDataType=uint16  BlockIOType=Outport  DeviceType=0
  out_OUT_PCAN.Tx_Ana.IN_ANA_08_SEL1_Sts.IN_ANA_Val : KIBES_Signal/KIBES_Signal  MBDS_LibraryBlock=on  DatabaseKey=2140  SignalName=OUT_PCAN.Tx_Ana.IN_ANA_08_SEL1_Sts.IN_ANA_Val  SymbolName=OUT_PCAN_Tx_Ana_IN_ANA_08_SEL1_Sts_IN_ANA_Val_002140  DataType=uint32  Init=0  Slope=1  Bias=0  DataSize=1  fpDataType=uint32  BlockIOType=Outport  DeviceType=0
  out_OUT_PCAN.Tx_Ana.IN_ANA_08_SEL1_Sts.MessageEnable : KIBES_Signal/KIBES_Signal  MBDS_LibraryBlock=on  DatabaseKey=2155  SignalName=OUT_PCAN.Tx_Ana.IN_ANA_08_SEL1_Sts.MessageEnable  SymbolName=OUT_PCAN_Tx_Ana_IN_ANA_08_SEL1_Sts_MessageEnable_002155  DataType=boolean  Init=0  Slope=1  Bias=0  DataSize=1  fpDataType=boolean  BlockIOType=Outport  DeviceType=0
  out_OUT_PCAN.Tx_Ana.IN_ANA_08_SEL2_Sts.IN_ANA_DIAG : KIBES_Signal/KIBES_Signal  MBDS_LibraryBlock=on  DatabaseKey=2141  SignalName=OUT_PCAN.Tx_Ana.IN_ANA_08_SEL2_Sts.IN_ANA_DIAG  SymbolName=OUT_PCAN_Tx_Ana_IN_ANA_08_SEL2_Sts_IN_ANA_DIAG_002141  DataType=uint16  Init=0  Slope=1  Bias=0  DataSize=1  fpDataType=uint16  BlockIOType=Outport  DeviceType=0
  out_OUT_PCAN.Tx_Ana.IN_ANA_08_SEL2_Sts.IN_ANA_Val : KIBES_Signal/KIBES_Signal  MBDS_LibraryBlock=on  DatabaseKey=2142  SignalName=OUT_PCAN.Tx_Ana.IN_ANA_08_SEL2_Sts.IN_ANA_Val  SymbolName=OUT_PCAN_Tx_Ana_IN_ANA_08_SEL2_Sts_IN_ANA_Val_002142  DataType=uint32  Init=0  Slope=1  Bias=0  DataSize=1  fpDataType=uint32  BlockIOType=Outport  DeviceType=0
  out_OUT_PCAN.Tx_Ana.IN_ANA_08_SEL2_Sts.MessageEnable : KIBES_Signal/KIBES_Signal  MBDS_LibraryBlock=on  DatabaseKey=2156  SignalName=OUT_PCAN.Tx_Ana.IN_ANA_08_SEL2_Sts.MessageEnable  SymbolName=OUT_PCAN_Tx_Ana_IN_ANA_08_SEL2_Sts_MessageEnable_002156  DataType=boolean  Init=0  Slope=1  Bias=0  DataSize=1  fpDataType=boolean  BlockIOType=Outport  DeviceType=0
  out_OUT_PCAN.Tx_Ana.IN_ANA_09_SEL1_Sts.IN_ANA_DIAG : KIBES_Signal/KIBES_Signal  MBDS_LibraryBlock=on  DatabaseKey=2143  SignalName=OUT_PCAN.Tx_Ana.IN_ANA_09_SEL1_Sts.IN_ANA_DIAG  SymbolName=OUT_PCAN_Tx_Ana_IN_ANA_09_SEL1_Sts_IN_ANA_DIAG_002143  DataType=uint16  Init=0  Slope=1  Bias=0  DataSize=1  fpDataType=uint16  BlockIOType=Outport  DeviceType=0
  out_OUT_PCAN.Tx_Ana.IN_ANA_09_SEL1_Sts.IN_ANA_Val : KIBES_Signal/KIBES_Signal  MBDS_LibraryBlock=on  DatabaseKey=2144  SignalName=OUT_PCAN.Tx_Ana.IN_ANA_09_SEL1_Sts.IN_ANA_Val  SymbolName=OUT_PCAN_Tx_Ana_IN_ANA_09_SEL1_Sts_IN_ANA_Val_002144  DataType=uint32  Init=0  Slope=1  Bias=0  DataSize=1  fpDataType=uint32  BlockIOType=Outport  DeviceType=0
  out_OUT_PCAN.Tx_Ana.IN_ANA_09_SEL1_Sts.MessageEnable : KIBES_Signal/KIBES_Signal  MBDS_LibraryBlock=on  DatabaseKey=2157  SignalName=OUT_PCAN.Tx_Ana.IN_ANA_09_SEL1_Sts.MessageEnable  SymbolName=OUT_PCAN_Tx_Ana_IN_ANA_09_SEL1_Sts_MessageEnable_002157  DataType=boolean  Init=0  Slope=1  Bias=0  DataSize=1  fpDataType=boolean  BlockIOType=Outport  DeviceType=0
  out_OUT_PCAN.Tx_Ana.IN_ANA_09_SEL2_Sts.IN_ANA_DIAG : KIBES_Signal/KIBES_Signal  MBDS_LibraryBlock=on  DatabaseKey=2145  SignalName=OUT_PCAN.Tx_Ana.IN_ANA_09_SEL2_Sts.IN_ANA_DIAG  SymbolName=OUT_PCAN_Tx_Ana_IN_ANA_09_SEL2_Sts_IN_ANA_DIAG_002145  DataType=uint16  Init=0  Slope=1  Bias=0  DataSize=1  fpDataType=uint16  BlockIOType=Outport  DeviceType=0
  out_OUT_PCAN.Tx_Ana.IN_ANA_09_SEL2_Sts.IN_ANA_Val : KIBES_Signal/KIBES_Signal  MBDS_LibraryBlock=on  DatabaseKey=2146  SignalName=OUT_PCAN.Tx_Ana.IN_ANA_09_SEL2_Sts.IN_ANA_Val  SymbolName=OUT_PCAN_Tx_Ana_IN_ANA_09_SEL2_Sts_IN_ANA_Val_002146  DataType=uint32  Init=0  Slope=1  Bias=0  DataSize=1  fpDataType=uint32  BlockIOType=Outport  DeviceType=0
  out_OUT_PCAN.Tx_Ana.IN_ANA_09_SEL2_Sts.MessageEnable : KIBES_Signal/KIBES_Signal  MBDS_LibraryBlock=on  DatabaseKey=2158  SignalName=OUT_PCAN.Tx_Ana.IN_ANA_09_SEL2_Sts.MessageEnable  SymbolName=OUT_PCAN_Tx_Ana_IN_ANA_09_SEL2_Sts_MessageEnable_002158  DataType=boolean  Init=0  Slope=1  Bias=0  DataSize=1  fpDataType=boolean  BlockIOType=Outport  DeviceType=0
  out_OUT_PCAN.Tx_Ana.IN_ANA_10_SEL1_Sts.IN_ANA_DIAG : KIBES_Signal/KIBES_Signal  MBDS_LibraryBlock=on  DatabaseKey=2147  SignalName=OUT_PCAN.Tx_Ana.IN_ANA_10_SEL1_Sts.IN_ANA_DIAG  SymbolName=OUT_PCAN_Tx_Ana_IN_ANA_10_SEL1_Sts_IN_ANA_DIAG_002147  DataType=uint16  Init=0  Slope=1  Bias=0  DataSize=1  fpDataType=uint16  BlockIOType=Outport  DeviceType=0
  out_OUT_PCAN.Tx_Ana.IN_ANA_10_SEL1_Sts.IN_ANA_Val : KIBES_Signal/KIBES_Signal  MBDS_LibraryBlock=on  DatabaseKey=2148  SignalName=OUT_PCAN.Tx_Ana.IN_ANA_10_SEL1_Sts.IN_ANA_Val  SymbolName=OUT_PCAN_Tx_Ana_IN_ANA_10_SEL1_Sts_IN_ANA_Val_002148  DataType=uint32  Init=0  Slope=1  Bias=0  DataSize=1  fpDataType=uint32  BlockIOType=Outport  DeviceType=0
  out_OUT_PCAN.Tx_Ana.IN_ANA_10_SEL1_Sts.MessageEnable : KIBES_Signal/KIBES_Signal  MBDS_LibraryBlock=on  DatabaseKey=2159  SignalName=OUT_PCAN.Tx_Ana.IN_ANA_10_SEL1_Sts.MessageEnable  SymbolName=OUT_PCAN_Tx_Ana_IN_ANA_10_SEL1_Sts_MessageEnable_002159  DataType=boolean  Init=0  Slope=1  Bias=0  DataSize=1  fpDataType=boolean  BlockIOType=Outport  DeviceType=0
  out_OUT_PCAN.Tx_Ana.IN_ANA_10_SEL2_Sts.IN_ANA_DIAG : KIBES_Signal/KIBES_Signal  MBDS_LibraryBlock=on  DatabaseKey=2149  SignalName=OUT_PCAN.Tx_Ana.IN_ANA_10_SEL2_Sts.IN_ANA_DIAG  SymbolName=OUT_PCAN_Tx_Ana_IN_ANA_10_SEL2_Sts_IN_ANA_DIAG_002149  DataType=uint16  Init=0  Slope=1  Bias=0  DataSize=1  fpDataType=uint16  BlockIOType=Outport  DeviceType=0
  out_OUT_PCAN.Tx_Ana.IN_ANA_10_SEL2_Sts.IN_ANA_Val : KIBES_Signal/KIBES_Signal  MBDS_LibraryBlock=on  DatabaseKey=2150  SignalName=OUT_PCAN.Tx_Ana.IN_ANA_10_SEL2_Sts.IN_ANA_Val  SymbolName=OUT_PCAN_Tx_Ana_IN_ANA_10_SEL2_Sts_IN_ANA_Val_002150  DataType=uint32  Init=0  Slope=1  Bias=0  DataSize=1  fpDataType=uint32  BlockIOType=Outport  DeviceType=0
  out_OUT_PCAN.Tx_Ana.IN_ANA_10_SEL2_Sts.MessageEnable : KIBES_Signal/KIBES_Signal  MBDS_LibraryBlock=on  DatabaseKey=2160  SignalName=OUT_PCAN.Tx_Ana.IN_ANA_10_SEL2_Sts.MessageEnable  SymbolName=OUT_PCAN_Tx_Ana_IN_ANA_10_SEL2_Sts_MessageEnable_002160  DataType=boolean  Init=0  Slope=1  Bias=0  DataSize=1  fpDataType=boolean  BlockIOType=Outport  DeviceType=0
  out_OUT_PCAN.Tx_Ana.IN_ANA_11_SEL1_Sts.IN_ANA_DIAG : KIBES_Signal/KIBES_Signal  MBDS_LibraryBlock=on  DatabaseKey=2151  SignalName=OUT_PCAN.Tx_Ana.IN_ANA_11_SEL1_Sts.IN_ANA_DIAG  SymbolName=OUT_PCAN_Tx_Ana_IN_ANA_11_SEL1_Sts_IN_ANA_DIAG_002151  DataType=uint16  Init=0  Slope=1  Bias=0  DataSize=1  fpDataType=uint16  BlockIOType=Outport  DeviceType=0
  out_OUT_PCAN.Tx_Ana.IN_ANA_11_SEL1_Sts.IN_ANA_Val : KIBES_Signal/KIBES_Signal  MBDS_LibraryBlock=on  DatabaseKey=2152  SignalName=OUT_PCAN.Tx_Ana.IN_ANA_11_SEL1_Sts.IN_ANA_Val  SymbolName=OUT_PCAN_Tx_Ana_IN_ANA_11_SEL1_Sts_IN_ANA_Val_002152  DataType=uint32  Init=0  Slope=1  Bias=0  DataSize=1  fpDataType=uint32  BlockIOType=Outport  DeviceType=0
  out_OUT_PCAN.Tx_Ana.IN_ANA_11_SEL1_Sts.MessageEnable : KIBES_Signal/KIBES_Signal  MBDS_LibraryBlock=on  DatabaseKey=2161  SignalName=OUT_PCAN.Tx_Ana.IN_ANA_11_SEL1_Sts.MessageEnable  SymbolName=OUT_PCAN_Tx_Ana_IN_ANA_11_SEL1_Sts_MessageEnable_002161  DataType=boolean  Init=0  Slope=1  Bias=0  DataSize=1  fpDataType=boolean  BlockIOType=Outport  DeviceType=0
  out_OUT_PCAN.Tx_Ana.IN_ANA_11_SEL2_Sts.IN_ANA_DIAG : KIBES_Signal/KIBES_Signal  MBDS_LibraryBlock=on  DatabaseKey=2153  SignalName=OUT_PCAN.Tx_Ana.IN_ANA_11_SEL2_Sts.IN_ANA_DIAG  SymbolName=OUT_PCAN_Tx_Ana_IN_ANA_11_SEL2_Sts_IN_ANA_DIAG_002153  DataType=uint16  Init=0  Slope=1  Bias=0  DataSize=1  fpDataType=uint16  BlockIOType=Outport  DeviceType=0
  out_OUT_PCAN.Tx_Ana.IN_ANA_11_SEL2_Sts.IN_ANA_Val : KIBES_Signal/KIBES_Signal  MBDS_LibraryBlock=on  DatabaseKey=2154  SignalName=OUT_PCAN.Tx_Ana.IN_ANA_11_SEL2_Sts.IN_ANA_Val  SymbolName=OUT_PCAN_Tx_Ana_IN_ANA_11_SEL2_Sts_IN_ANA_Val_002154  DataType=uint32  Init=0  Slope=1  Bias=0  DataSize=1  fpDataType=uint32  BlockIOType=Outport  DeviceType=0
  out_OUT_PCAN.Tx_Ana.IN_ANA_11_SEL2_Sts.MessageEnable : KIBES_Signal/KIBES_Signal  MBDS_LibraryBlock=on  DatabaseKey=2162  SignalName=OUT_PCAN.Tx_Ana.IN_ANA_11_SEL2_Sts.MessageEnable  SymbolName=OUT_PCAN_Tx_Ana_IN_ANA_11_SEL2_Sts_MessageEnable_002162  DataType=boolean  Init=0  Slope=1  Bias=0  DataSize=1  fpDataType=boolean  BlockIOType=Outport  DeviceType=0
  out_OUT_PCAN.Tx_Ana.In_Ana_01_Sts.IN_ANA_DIAG : KIBES_Signal/KIBES_Signal  MBDS_LibraryBlock=on  DatabaseKey=1718  SignalName=OUT_PCAN.Tx_Ana.In_Ana_01_Sts.IN_ANA_DIAG  SymbolName=OUT_PCAN_Tx_Ana_In_Ana_01_Sts_IN_ANA_DIAG_001718  DataType=uint16  Init=0  Slope=1  Bias=0  DataSize=1  fpDataType=uint16  BlockIOType=Outport  DeviceType=0
  out_OUT_PCAN.Tx_Ana.In_Ana_01_Sts.IN_ANA_Val : KIBES_Signal/KIBES_Signal  MBDS_LibraryBlock=on  DatabaseKey=1719  SignalName=OUT_PCAN.Tx_Ana.In_Ana_01_Sts.IN_ANA_Val  SymbolName=OUT_PCAN_Tx_Ana_In_Ana_01_Sts_IN_ANA_Val_001719  DataType=uint32  Init=0  Slope=1  Bias=0  DataSize=1  fpDataType=uint32  BlockIOType=Outport  DeviceType=0
  out_OUT_PCAN.Tx_Ana.In_Ana_01_Sts.MessageEnable : KIBES_Signal/KIBES_Signal  MBDS_LibraryBlock=on  DatabaseKey=1748  SignalName=OUT_PCAN.Tx_Ana.In_Ana_01_Sts.MessageEnable  SymbolName=OUT_PCAN_Tx_Ana_In_Ana_01_Sts_MessageEnable_001748  DataType=boolean  Init=0  Slope=1  Bias=0  DataSize=1  fpDataType=boolean  BlockIOType=Outport  DeviceType=0
  out_OUT_PCAN.Tx_Ana.In_Ana_02_Sts.IN_ANA_DIAG : KIBES_Signal/KIBES_Signal  MBDS_LibraryBlock=on  DatabaseKey=1720  SignalName=OUT_PCAN.Tx_Ana.In_Ana_02_Sts.IN_ANA_DIAG  SymbolName=OUT_PCAN_Tx_Ana_In_Ana_02_Sts_IN_ANA_DIAG_001720  DataType=uint16  Init=0  Slope=1  Bias=0  DataSize=1  fpDataType=uint16  BlockIOType=Outport  DeviceType=0
  out_OUT_PCAN.Tx_Ana.In_Ana_02_Sts.IN_ANA_Val : KIBES_Signal/KIBES_Signal  MBDS_LibraryBlock=on  DatabaseKey=1721  SignalName=OUT_PCAN.Tx_Ana.In_Ana_02_Sts.IN_ANA_Val  SymbolName=OUT_PCAN_Tx_Ana_In_Ana_02_Sts_IN_ANA_Val_001721  DataType=uint32  Init=0  Slope=1  Bias=0  DataSize=1  fpDataType=uint32  BlockIOType=Outport  DeviceType=0
  out_OUT_PCAN.Tx_Ana.In_Ana_02_Sts.MessageEnable : KIBES_Signal/KIBES_Signal  MBDS_LibraryBlock=on  DatabaseKey=1749  SignalName=OUT_PCAN.Tx_Ana.In_Ana_02_Sts.MessageEnable  SymbolName=OUT_PCAN_Tx_Ana_In_Ana_02_Sts_MessageEnable_001749  DataType=boolean  Init=0  Slope=1  Bias=0  DataSize=1  fpDataType=boolean  BlockIOType=Outport  DeviceType=0
  out_OUT_PCAN.Tx_Ana.In_Ana_03_Sts.IN_ANA_DIAG : KIBES_Signal/KIBES_Signal  MBDS_LibraryBlock=on  DatabaseKey=1722  SignalName=OUT_PCAN.Tx_Ana.In_Ana_03_Sts.IN_ANA_DIAG  SymbolName=OUT_PCAN_Tx_Ana_In_Ana_03_Sts_IN_ANA_DIAG_001722  DataType=uint16  Init=0  Slope=1  Bias=0  DataSize=1  fpDataType=uint16  BlockIOType=Outport  DeviceType=0
  out_OUT_PCAN.Tx_Ana.In_Ana_03_Sts.IN_ANA_Val : KIBES_Signal/KIBES_Signal  MBDS_LibraryBlock=on  DatabaseKey=1723  SignalName=OUT_PCAN.Tx_Ana.In_Ana_03_Sts.IN_ANA_Val  SymbolName=OUT_PCAN_Tx_Ana_In_Ana_03_Sts_IN_ANA_Val_001723  DataType=uint32  Init=0  Slope=1  Bias=0  DataSize=1  fpDataType=uint32  BlockIOType=Outport  DeviceType=0
  out_OUT_PCAN.Tx_Ana.In_Ana_03_Sts.MessageEnable : KIBES_Signal/KIBES_Signal  MBDS_LibraryBlock=on  DatabaseKey=1750  SignalName=OUT_PCAN.Tx_Ana.In_Ana_03_Sts.MessageEnable  SymbolName=OUT_PCAN_Tx_Ana_In_Ana_03_Sts_MessageEnable_001750  DataType=boolean  Init=0  Slope=1  Bias=0  DataSize=1  fpDataType=boolean  BlockIOType=Outport  DeviceType=0
  out_OUT_PCAN.Tx_Ana.In_Ana_04_Sts.IN_ANA_DIAG : KIBES_Signal/KIBES_Signal  MBDS_LibraryBlock=on  DatabaseKey=1724  SignalName=OUT_PCAN.Tx_Ana.In_Ana_04_Sts.IN_ANA_DIAG  SymbolName=OUT_PCAN_Tx_Ana_In_Ana_04_Sts_IN_ANA_DIAG_001724  DataType=uint16  Init=0  Slope=1  Bias=0  DataSize=1  fpDataType=uint16  BlockIOType=Outport  DeviceType=0
  out_OUT_PCAN.Tx_Ana.In_Ana_04_Sts.IN_ANA_Val : KIBES_Signal/KIBES_Signal  MBDS_LibraryBlock=on  DatabaseKey=1725  SignalName=OUT_PCAN.Tx_Ana.In_Ana_04_Sts.IN_ANA_Val  SymbolName=OUT_PCAN_Tx_Ana_In_Ana_04_Sts_IN_ANA_Val_001725  DataType=uint32  Init=0  Slope=1  Bias=0  DataSize=1  fpDataType=uint32  BlockIOType=Outport  DeviceType=0
  out_OUT_PCAN.Tx_Ana.In_Ana_04_Sts.MessageEnable : KIBES_Signal/KIBES_Signal  MBDS_LibraryBlock=on  DatabaseKey=1751  SignalName=OUT_PCAN.Tx_Ana.In_Ana_04_Sts.MessageEnable  SymbolName=OUT_PCAN_Tx_Ana_In_Ana_04_Sts_MessageEnable_001751  DataType=boolean  Init=0  Slope=1  Bias=0  DataSize=1  fpDataType=boolean  BlockIOType=Outport  DeviceType=0
  out_OUT_PCAN.Tx_Ana.In_Ana_05_Sts.IN_ANA_DIAG : KIBES_Signal/KIBES_Signal  MBDS_LibraryBlock=on  DatabaseKey=1726  SignalName=OUT_PCAN.Tx_Ana.In_Ana_05_Sts.IN_ANA_DIAG  SymbolName=OUT_PCAN_Tx_Ana_In_Ana_05_Sts_IN_ANA_DIAG_001726  DataType=uint16  Init=0  Slope=1  Bias=0  DataSize=1  fpDataType=uint16  BlockIOType=Outport  DeviceType=0
  out_OUT_PCAN.Tx_Ana.In_Ana_05_Sts.IN_ANA_Val : KIBES_Signal/KIBES_Signal  MBDS_LibraryBlock=on  DatabaseKey=1727  SignalName=OUT_PCAN.Tx_Ana.In_Ana_05_Sts.IN_ANA_Val  SymbolName=OUT_PCAN_Tx_Ana_In_Ana_05_Sts_IN_ANA_Val_001727  DataType=uint32  Init=0  Slope=1  Bias=0  DataSize=1  fpDataType=uint32  BlockIOType=Outport  DeviceType=0
  out_OUT_PCAN.Tx_Ana.In_Ana_05_Sts.MessageEnable : KIBES_Signal/KIBES_Signal  MBDS_LibraryBlock=on  DatabaseKey=1752  SignalName=OUT_PCAN.Tx_Ana.In_Ana_05_Sts.MessageEnable  SymbolName=OUT_PCAN_Tx_Ana_In_Ana_05_Sts_MessageEnable_001752  DataType=boolean  Init=0  Slope=1  Bias=0  DataSize=1  fpDataType=boolean  BlockIOType=Outport  DeviceType=0
  out_OUT_PCAN.Tx_Ana.In_Ana_06_Sts.IN_ANA_DIAG : KIBES_Signal/KIBES_Signal  MBDS_LibraryBlock=on  DatabaseKey=1728  SignalName=OUT_PCAN.Tx_Ana.In_Ana_06_Sts.IN_ANA_DIAG  SymbolName=OUT_PCAN_Tx_Ana_In_Ana_06_Sts_IN_ANA_DIAG_001728  DataType=uint16  Init=0  Slope=1  Bias=0  DataSize=1  fpDataType=uint16  BlockIOType=Outport  DeviceType=0
  out_OUT_PCAN.Tx_Ana.In_Ana_06_Sts.IN_ANA_Val : KIBES_Signal/KIBES_Signal  MBDS_LibraryBlock=on  DatabaseKey=1729  SignalName=OUT_PCAN.Tx_Ana.In_Ana_06_Sts.IN_ANA_Val  SymbolName=OUT_PCAN_Tx_Ana_In_Ana_06_Sts_IN_ANA_Val_001729  DataType=uint32  Init=0  Slope=1  Bias=0  DataSize=1  fpDataType=uint32  BlockIOType=Outport  DeviceType=0
  out_OUT_PCAN.Tx_Ana.In_Ana_06_Sts.MessageEnable : KIBES_Signal/KIBES_Signal  MBDS_LibraryBlock=on  DatabaseKey=1753  SignalName=OUT_PCAN.Tx_Ana.In_Ana_06_Sts.MessageEnable  SymbolName=OUT_PCAN_Tx_Ana_In_Ana_06_Sts_MessageEnable_001753  DataType=boolean  Init=0  Slope=1  Bias=0  DataSize=1  fpDataType=boolean  BlockIOType=Outport  DeviceType=0
  out_OUT_PCAN.Tx_Ana.In_Ana_07_Sts.IN_ANA_DIAG : KIBES_Signal/KIBES_Signal  MBDS_LibraryBlock=on  DatabaseKey=1730  SignalName=OUT_PCAN.Tx_Ana.In_Ana_07_Sts.IN_ANA_DIAG  SymbolName=OUT_PCAN_Tx_Ana_In_Ana_07_Sts_IN_ANA_DIAG_001730  DataType=uint16  Init=0  Slope=1  Bias=0  DataSize=1  fpDataType=uint16  BlockIOType=Outport  DeviceType=0
  out_OUT_PCAN.Tx_Ana.In_Ana_07_Sts.IN_ANA_Val : KIBES_Signal/KIBES_Signal  MBDS_LibraryBlock=on  DatabaseKey=1731  SignalName=OUT_PCAN.Tx_Ana.In_Ana_07_Sts.IN_ANA_Val  SymbolName=OUT_PCAN_Tx_Ana_In_Ana_07_Sts_IN_ANA_Val_001731  DataType=uint32  Init=0  Slope=1  Bias=0  DataSize=1  fpDataType=uint32  BlockIOType=Outport  DeviceType=0
  out_OUT_PCAN.Tx_Ana.In_Ana_07_Sts.MessageEnable : KIBES_Signal/KIBES_Signal  MBDS_LibraryBlock=on  DatabaseKey=1754  SignalName=OUT_PCAN.Tx_Ana.In_Ana_07_Sts.MessageEnable  SymbolName=OUT_PCAN_Tx_Ana_In_Ana_07_Sts_MessageEnable_001754  DataType=boolean  Init=0  Slope=1  Bias=0  DataSize=1  fpDataType=boolean  BlockIOType=Outport  DeviceType=0
  out_OUT_PCAN.Tx_Ana.In_Ana_12_Sts.IN_ANA_DIAG : KIBES_Signal/KIBES_Signal  MBDS_LibraryBlock=on  DatabaseKey=1740  SignalName=OUT_PCAN.Tx_Ana.In_Ana_12_Sts.IN_ANA_DIAG  SymbolName=OUT_PCAN_Tx_Ana_In_Ana_12_Sts_IN_ANA_DIAG_001740  DataType=uint16  Init=0  Slope=1  Bias=0  DataSize=1  fpDataType=uint16  BlockIOType=Outport  DeviceType=0
  out_OUT_PCAN.Tx_Ana.In_Ana_12_Sts.IN_ANA_Val : KIBES_Signal/KIBES_Signal  MBDS_LibraryBlock=on  DatabaseKey=1741  SignalName=OUT_PCAN.Tx_Ana.In_Ana_12_Sts.IN_ANA_Val  SymbolName=OUT_PCAN_Tx_Ana_In_Ana_12_Sts_IN_ANA_Val_001741  DataType=uint32  Init=0  Slope=1  Bias=0  DataSize=1  fpDataType=uint32  BlockIOType=Outport  DeviceType=0
  out_OUT_PCAN.Tx_Ana.In_Ana_12_Sts.MessageEnable : KIBES_Signal/KIBES_Signal  MBDS_LibraryBlock=on  DatabaseKey=1759  SignalName=OUT_PCAN.Tx_Ana.In_Ana_12_Sts.MessageEnable  SymbolName=OUT_PCAN_Tx_Ana_In_Ana_12_Sts_MessageEnable_001759  DataType=boolean  Init=0  Slope=1  Bias=0  DataSize=1  fpDataType=boolean  BlockIOType=Outport  DeviceType=0
  out_OUT_PCAN.Tx_Ana.In_Ana_13_Sts.IN_ANA_DIAG : KIBES_Signal/KIBES_Signal  MBDS_LibraryBlock=on  DatabaseKey=1742  SignalName=OUT_PCAN.Tx_Ana.In_Ana_13_Sts.IN_ANA_DIAG  SymbolName=OUT_PCAN_Tx_Ana_In_Ana_13_Sts_IN_ANA_DIAG_001742  DataType=uint16  Init=0  Slope=1  Bias=0  DataSize=1  fpDataType=uint16  BlockIOType=Outport  DeviceType=0
  out_OUT_PCAN.Tx_Ana.In_Ana_13_Sts.IN_ANA_Val : KIBES_Signal/KIBES_Signal  MBDS_LibraryBlock=on  DatabaseKey=1743  SignalName=OUT_PCAN.Tx_Ana.In_Ana_13_Sts.IN_ANA_Val  SymbolName=OUT_PCAN_Tx_Ana_In_Ana_13_Sts_IN_ANA_Val_001743  DataType=uint32  Init=0  Slope=1  Bias=0  DataSize=1  fpDataType=uint32  BlockIOType=Outport  DeviceType=0
  out_OUT_PCAN.Tx_Ana.In_Ana_13_Sts.MessageEnable : KIBES_Signal/KIBES_Signal  MBDS_LibraryBlock=on  DatabaseKey=1760  SignalName=OUT_PCAN.Tx_Ana.In_Ana_13_Sts.MessageEnable  SymbolName=OUT_PCAN_Tx_Ana_In_Ana_13_Sts_MessageEnable_001760  DataType=boolean  Init=0  Slope=1  Bias=0  DataSize=1  fpDataType=boolean  BlockIOType=Outport  DeviceType=0
  out_OUT_PCAN.Tx_Ana.In_Ana_14_Sts.IN_ANA_DIAG : KIBES_Signal/KIBES_Signal  MBDS_LibraryBlock=on  DatabaseKey=1744  SignalName=OUT_PCAN.Tx_Ana.In_Ana_14_Sts.IN_ANA_DIAG  SymbolName=OUT_PCAN_Tx_Ana_In_Ana_14_Sts_IN_ANA_DIAG_001744  DataType=uint16  Init=0  Slope=1  Bias=0  DataSize=1  fpDataType=uint16  BlockIOType=Outport  DeviceType=0
  out_OUT_PCAN.Tx_Ana.In_Ana_14_Sts.IN_ANA_Val : KIBES_Signal/KIBES_Signal  MBDS_LibraryBlock=on  DatabaseKey=1745  SignalName=OUT_PCAN.Tx_Ana.In_Ana_14_Sts.IN_ANA_Val  SymbolName=OUT_PCAN_Tx_Ana_In_Ana_14_Sts_IN_ANA_Val_001745  DataType=uint32  Init=0  Slope=1  Bias=0  DataSize=1  fpDataType=uint32  BlockIOType=Outport  DeviceType=0
  out_OUT_PCAN.Tx_Ana.In_Ana_14_Sts.MessageEnable : KIBES_Signal/KIBES_Signal  MBDS_LibraryBlock=on  DatabaseKey=1761  SignalName=OUT_PCAN.Tx_Ana.In_Ana_14_Sts.MessageEnable  SymbolName=OUT_PCAN_Tx_Ana_In_Ana_14_Sts_MessageEnable_001761  DataType=boolean  Init=0  Slope=1  Bias=0  DataSize=1  fpDataType=boolean  BlockIOType=Outport  DeviceType=0
  out_OUT_PCAN.Tx_Ana.In_Ana_15_Sts.IN_ANA_DIAG : KIBES_Signal/KIBES_Signal  MBDS_LibraryBlock=on  DatabaseKey=1746  SignalName=OUT_PCAN.Tx_Ana.In_Ana_15_Sts.IN_ANA_DIAG  SymbolName=OUT_PCAN_Tx_Ana_In_Ana_15_Sts_IN_ANA_DIAG_001746  DataType=uint16  Init=0  Slope=1  Bias=0  DataSize=1  fpDataType=uint16  BlockIOType=Outport  DeviceType=0
  out_OUT_PCAN.Tx_Ana.In_Ana_15_Sts.IN_ANA_Val : KIBES_Signal/KIBES_Signal  MBDS_LibraryBlock=on  DatabaseKey=1747  SignalName=OUT_PCAN.Tx_Ana.In_Ana_15_Sts.IN_ANA_Val  SymbolName=OUT_PCAN_Tx_Ana_In_Ana_15_Sts_IN_ANA_Val_001747  DataType=uint32  Init=0  Slope=1  Bias=0  DataSize=1  fpDataType=uint32  BlockIOType=Outport  DeviceType=0
  out_OUT_PCAN.Tx_Ana.In_Ana_15_Sts.MessageEnable : KIBES_Signal/KIBES_Signal  MBDS_LibraryBlock=on  DatabaseKey=1762  SignalName=OUT_PCAN.Tx_Ana.In_Ana_15_Sts.MessageEnable  SymbolName=OUT_PCAN_Tx_Ana_In_Ana_15_Sts_MessageEnable_001762  DataType=boolean  Init=0  Slope=1  Bias=0  DataSize=1  fpDataType=boolean  BlockIOType=Outport  DeviceType=0
  wires:
  bo_SendEnable/1 -> out_OUT_PCAN.Tx_Ana.In_Ana_01_Sts.MessageEnable/1, out_OUT_PCAN.Tx_Ana.In_Ana_02_Sts.MessageEnable/1, out_OUT_PCAN.Tx_Ana.In_Ana_03_Sts.MessageEnable/1, out_OUT_PCAN.Tx_Ana.In_Ana_04_Sts.MessageEnable/1, out_OUT_PCAN.Tx_Ana.In_Ana_05_Sts.MessageEnable/1, out_OUT_PCAN.Tx_Ana.In_Ana_06_Sts.MessageEnable/1, out_OUT_PCAN.Tx_Ana.In_Ana_07_Sts.MessageEnable/1, out_OUT_PCAN.Tx_Ana.IN_ANA_08_SEL1_Sts.MessageEnable/1, out_OUT_PCAN.Tx_Ana.IN_ANA_08_SEL2_Sts.MessageEnable/1, out_OUT_PCAN.Tx_Ana.IN_ANA_09_SEL2_Sts.MessageEnable/1, out_OUT_PCAN.Tx_Ana.IN_ANA_10_SEL1_Sts.MessageEnable/1, out_OUT_PCAN.Tx_Ana.In_Ana_12_Sts.MessageEnable/1, out_OUT_PCAN.Tx_Ana.In_Ana_13_Sts.MessageEnable/1, out_OUT_PCAN.Tx_Ana.In_Ana_15_Sts.MessageEnable/1, out_OUT_PCAN.Tx_Ana.In_Ana_14_Sts.MessageEnable/1, out_OUT_PCAN.Tx_Ana.IN_ANA_11_SEL2_Sts.MessageEnable/1, out_OUT_PCAN.Tx_Ana.IN_ANA_11_SEL1_Sts.MessageEnable/1, out_OUT_PCAN.Tx_Ana.IN_ANA_10_SEL2_Sts.MessageEnable/1, out_OUT_PCAN.Tx_Ana.IN_ANA_09_SEL1_Sts.MessageEnable/1
  in_DIAG_AnalogInputs.IN_ANA_07_DIAG/1 -> out_OUT_PCAN.Tx_Ana.In_Ana_07_Sts.IN_ANA_DIAG/1
  in_IN_AnalogInputs.IN_ANA_11_SEL1/1 -> out_OUT_PCAN.Tx_Ana.IN_ANA_11_SEL1_Sts.IN_ANA_Val/1
  in_DIAG_AnalogInputs.IN_ANA_01_DIAG/1 -> out_OUT_PCAN.Tx_Ana.In_Ana_01_Sts.IN_ANA_DIAG/1
  in_IN_AnalogInputs.IN_ANA_09_SEL1/1 -> out_OUT_PCAN.Tx_Ana.IN_ANA_09_SEL1_Sts.IN_ANA_Val/1
  in_IN_AnalogInputs.IN_ANA_07/1 -> out_OUT_PCAN.Tx_Ana.In_Ana_07_Sts.IN_ANA_Val/1
  in_DIAG_AnalogInputs.IN_ANA_11_SEL1_DIAG/1 -> out_OUT_PCAN.Tx_Ana.IN_ANA_11_SEL1_Sts.IN_ANA_DIAG/1
  in_DIAG_AnalogInputs.IN_ANA_02_DIAG/1 -> out_OUT_PCAN.Tx_Ana.In_Ana_02_Sts.IN_ANA_DIAG/1
  in_IN_AnalogInputs.IN_ANA_04/1 -> out_OUT_PCAN.Tx_Ana.In_Ana_04_Sts.IN_ANA_Val/1
  in_DIAG_AnalogInputs.IN_ANA_08_SEL1_DIAG/1 -> out_OUT_PCAN.Tx_Ana.IN_ANA_08_SEL1_Sts.IN_ANA_DIAG/1
  in_IN_AnalogInputs.IN_ANA_08_SEL1/1 -> out_OUT_PCAN.Tx_Ana.IN_ANA_08_SEL1_Sts.IN_ANA_Val/1
  in_IN_AnalogInputs.IN_ANA_03/1 -> out_OUT_PCAN.Tx_Ana.In_Ana_03_Sts.IN_ANA_Val/1
  in_IN_AnalogInputs.IN_ANA_05/1 -> out_OUT_PCAN.Tx_Ana.In_Ana_05_Sts.IN_ANA_Val/1
  in_DIAG_AnalogInputs.IN_ANA_05_DIAG/1 -> out_OUT_PCAN.Tx_Ana.In_Ana_05_Sts.IN_ANA_DIAG/1
  in_IN_AnalogInputs.IN_ANA_06/1 -> out_OUT_PCAN.Tx_Ana.In_Ana_06_Sts.IN_ANA_Val/1
  in_DIAG_AnalogInputs.IN_ANA_06_DIAG/1 -> out_OUT_PCAN.Tx_Ana.In_Ana_06_Sts.IN_ANA_DIAG/1
  in_DIAG_AnalogInputs.IN_ANA_04_DIAG/1 -> out_OUT_PCAN.Tx_Ana.In_Ana_04_Sts.IN_ANA_DIAG/1
  in_DIAG_AnalogInputs.IN_ANA_09_SEL1_DIAG/1 -> out_OUT_PCAN.Tx_Ana.IN_ANA_09_SEL1_Sts.IN_ANA_DIAG/1
  in_IN_AnalogInputs.IN_ANA_01/1 -> out_OUT_PCAN.Tx_Ana.In_Ana_01_Sts.IN_ANA_Val/1
  in_IN_AnalogInputs.IN_ANA_02/1 -> out_OUT_PCAN.Tx_Ana.In_Ana_02_Sts.IN_ANA_Val/1
  in_DIAG_AnalogInputs.IN_ANA_03_DIAG/1 -> out_OUT_PCAN.Tx_Ana.In_Ana_03_Sts.IN_ANA_DIAG/1
  in_DIAG_AnalogInputs.IN_ANA_10_SEL1_DIAG/1 -> out_OUT_PCAN.Tx_Ana.IN_ANA_10_SEL1_Sts.IN_ANA_DIAG/1
  in_IN_AnalogInputs.IN_ANA_10_SEL1/1 -> out_OUT_PCAN.Tx_Ana.IN_ANA_10_SEL1_Sts.IN_ANA_Val/1
  in_IN_AnalogInputsCoolant.IN_ANA_12/1 -> out_OUT_PCAN.Tx_Ana.In_Ana_12_Sts.IN_ANA_Val/1
  in_DIAG_AnalogInputsCoolant.IN_ANA_12_DIAG/1 -> out_OUT_PCAN.Tx_Ana.In_Ana_12_Sts.IN_ANA_DIAG/1
  in_IN_AnalogInputsCoolant.IN_ANA_13/1 -> out_OUT_PCAN.Tx_Ana.In_Ana_13_Sts.IN_ANA_Val/1
  in_DIAG_AnalogInputsCoolant.IN_ANA_13_DIAG/1 -> out_OUT_PCAN.Tx_Ana.In_Ana_13_Sts.IN_ANA_DIAG/1
  in_IN_AnalogInputs.OUT_FREQ_feedback.IN_ANA_14/1 -> out_OUT_PCAN.Tx_Ana.In_Ana_14_Sts.IN_ANA_Val/1
  in_DIAG_AnalogInputs.OUT_FREQ_feedback.IN_ANA_14_DIAG/1 -> out_OUT_PCAN.Tx_Ana.In_Ana_14_Sts.IN_ANA_DIAG/1
  in_IN_AnalogInputs.OUT_FREQ_feedback.IN_ANA_15/1 -> out_OUT_PCAN.Tx_Ana.In_Ana_15_Sts.IN_ANA_Val/1
  in_DIAG_AnalogInputs.OUT_FREQ_feedback.IN_ANA_15_DIAG/1 -> out_OUT_PCAN.Tx_Ana.In_Ana_15_Sts.IN_ANA_DIAG/1
  in_IN_AnalogInputs.IN_ANA_08_SEL2/1 -> out_OUT_PCAN.Tx_Ana.IN_ANA_08_SEL2_Sts.IN_ANA_Val/1
  in_DIAG_AnalogInputs.IN_ANA_08_SEL2_DIAG/1 -> out_OUT_PCAN.Tx_Ana.IN_ANA_08_SEL2_Sts.IN_ANA_DIAG/1
  in_IN_AnalogInputs.IN_ANA_09_SEL2/1 -> out_OUT_PCAN.Tx_Ana.IN_ANA_09_SEL2_Sts.IN_ANA_Val/1
  in_DIAG_AnalogInputs.IN_ANA_09_SEL2_DIAG/1 -> out_OUT_PCAN.Tx_Ana.IN_ANA_09_SEL2_Sts.IN_ANA_DIAG/1
  in_IN_AnalogInputs.IN_ANA_10_SEL2/1 -> out_OUT_PCAN.Tx_Ana.IN_ANA_10_SEL2_Sts.IN_ANA_Val/1
  in_DIAG_AnalogInputs.IN_ANA_10_SEL2_DIAG/1 -> out_OUT_PCAN.Tx_Ana.IN_ANA_10_SEL2_Sts.IN_ANA_DIAG/1
  in_IN_AnalogInputs.IN_ANA_11_SEL2/1 -> out_OUT_PCAN.Tx_Ana.IN_ANA_11_SEL2_Sts.IN_ANA_Val/1
  in_DIAG_AnalogInputs.IN_ANA_11_SEL2_DIAG/1 -> out_OUT_PCAN.Tx_Ana.IN_ANA_11_SEL2_Sts.IN_ANA_DIAG/1
  Constant/1 -> out_OUT_PCAN.Rx_Ctrl.In_Ana_Ctrl.MessageEnable/1
  in_IN_PCAN.Rx_Ctrl.In_Ana_Ctrl.MessageState/1 -> EQ/1(u1)
  Constant1/1 -> EQ/2(u2)
  EQ/1(y) -> [boCtrlValid]
  [boCtrlValid] -> AND3/1(u1), AND2/1(u1), AND1/1(u1), AND/1(u1)
  in_IN_PCAN.Rx_Ctrl.In_Ana_Ctrl.IN_ANA_08_SWT1/1 -> AND/2(u2)
  AND/1(y) -> out_OUT_DigitalOutputsSTATIC.IN_ANA_08_SWT1/1
  AND1/1(y) -> out_OUT_DigitalOutputsSTATIC.IN_ANA_09_SWT1/1
  AND2/1(y) -> out_OUT_DigitalOutputsSTATIC.IN_ANA_10_SWT1/1
  AND3/1(y) -> out_OUT_DigitalOutputsSTATIC.IN_ANA_11_SWT1/1
  in_IN_PCAN.Rx_Ctrl.In_Ana_Ctrl.IN_ANA_09_SWT1/1 -> AND1/2(u2)
  in_IN_PCAN.Rx_Ctrl.In_Ana_Ctrl.IN_ANA_10_SWT1/1 -> AND2/2(u2)
  in_IN_PCAN.Rx_Ctrl.In_Ana_Ctrl.IN_ANA_11_SWT1/1 -> AND3/2(u2)
